simulink model "Q_3"  (R2020a)
settings: Solver=VariableStepAuto  StartTime=0.0  StopTime=10.0  RelTol=1e-3
undefined symbols (not defined in the file): b, Ki, Kp, m
settings Model: DataDictionary=CruiseDD.sldd  Creator=Admin  LastModifiedBy=Admin

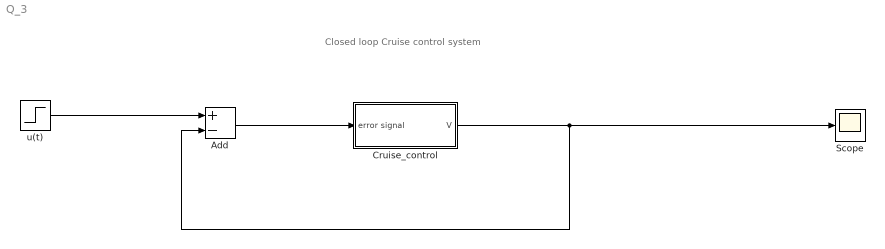
== system Q_3 ==
  note: Closed loop Cruise control system
  Add : Sum  Inputs=+-
  Cruise_control : Subsystem  TreatAsAtomicUnit=on
  Scope : Scope
  u(t) : Step  After=u  SampleTime=0
  wires:
  u(t)/1 -> Add/1
  Add/1 -> Cruise_control/1(error signal)
  Cruise_control/1(V) -> Add/2, Scope/1

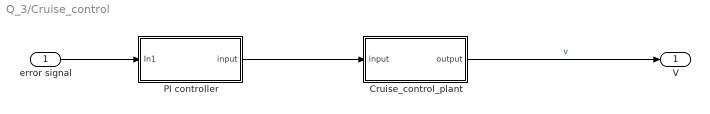
== system Q_3/Cruise_control ==
  error signal : Inport
  Cruise_control_plant : Subsystem  TreatAsAtomicUnit=on
  PI controller : Subsystem  TreatAsAtomicUnit=on
  V : Outport
  wires:
  PI controller/1(input) -> Cruise_control_plant/1(input)
  Cruise_control_plant/1(output) -> V/1  "v"
  error signal/1 -> PI controller/1(In1)

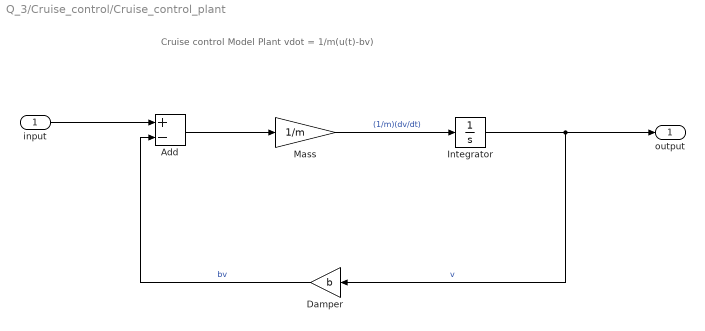
== system Q_3/Cruise_control/Cruise_control_plant ==
  note: Cruise control Model Plant
      | vdot = 1/m(u(t)-bv)
  input : Inport
  Add : Sum  Inputs=+-
  Damper : Gain  Gain=b
  Integrator : Integrator
  Mass : Gain  Gain=1/m
  output : Outport
  wires:
  Mass/1 -> Integrator/1  "(1/m)(dv/dt)"
  Integrator/1 -> Damper/1, output/1  "v"
  Add/1 -> Mass/1
  Damper/1 -> Add/2  "bv"
  input/1 -> Add/1

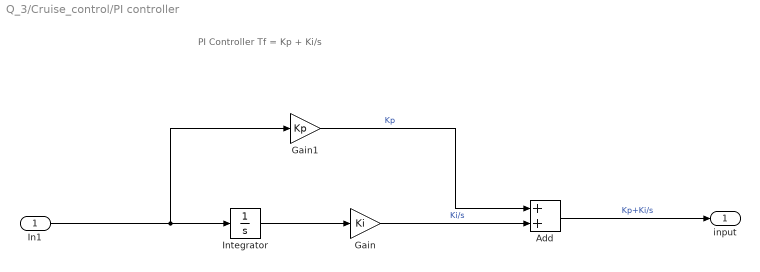
== system Q_3/Cruise_control/PI controller ==
  note: PI Controller
      | Tf = Kp + Ki/s
  In1 : Inport
  Add : Sum
  Gain : Gain  Gain=Ki
  Gain1 : Gain  Gain=Kp
  Integrator : Integrator
  input : Outport
  wires:
  Gain1/1 -> Add/1  "Kp"
  In1/1 -> Integrator/1, Gain1/1
  Add/1 -> input/1  "Kp+Ki/s"
  Gain/1 -> Add/2  "Ki/s"
  Integrator/1 -> Gain/1
